simulink model "UFR_Monitoring_System"  (R2023a)
settings: Solver=VariableStepAuto  StartTime=0.0  StopTime=3600*4  RelTol=1e-3
undefined symbols (not defined in the file): out
settings Model: PacingRate=0.100000  Creator=alibacon  LastModifiedBy=ppatel
settings DataIOCC: SaveOutput=off  SaveTime=off
settings DebuggingCC: SubsystemReferenceDiagnosticForUnitTest=warning

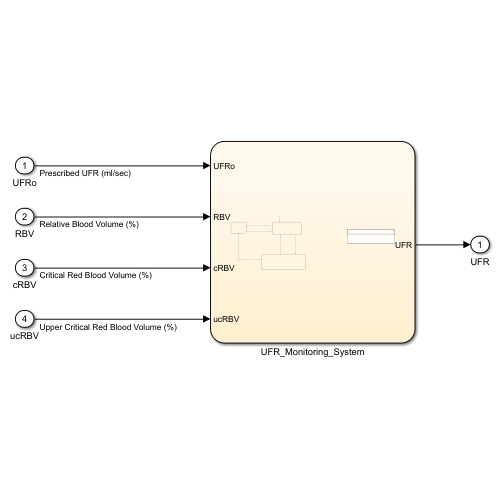
[thumbnail: Simulink's stored preview of the top-level diagram]
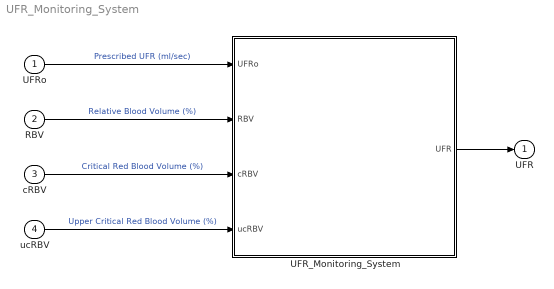
== system UFR_Monitoring_System ==
  UFRo : Inport  OutDataTypeStr=double  PortDimensions=1
  RBV : Inport  Port=2  OutDataTypeStr=double  PortDimensions=1  SampleTime=0
  cRBV : Inport  Port=3  OutDataTypeStr=double  PortDimensions=1  SampleTime=[0,1]
  ucRBV : Inport  Port=4  OutDataTypeStr=double  PortDimensions=1  SampleTime=[0,1]
  UFR_Monitoring_System : Stateflow chart  TreatAsAtomicUnit=on
  UFR : Outport  OutDataTypeStr=double  PortDimensions=1  SampleTime=[0,1]
  wires:
  UFRo/1 -> UFR_Monitoring_System/1(UFRo)  "Prescribed UFR (ml/sec)"
  RBV/1 -> UFR_Monitoring_System/2(RBV)  "Relative Blood Volume (%)"
  cRBV/1 -> UFR_Monitoring_System/3(cRBV)  "Critical Red Blood Volume (%)"
  ucRBV/1 -> UFR_Monitoring_System/4(ucRBV)  "Upper Critical Red Blood Volume (%)"
  UFR_Monitoring_System/1(UFR) -> UFR/1

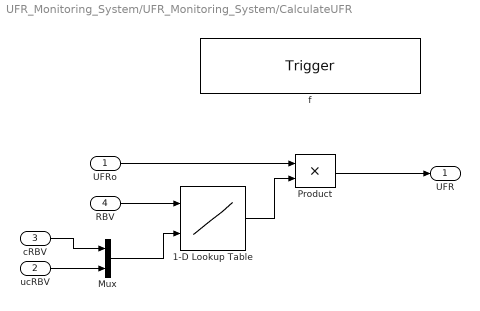
== system UFR_Monitoring_System/UFR_Monitoring_System/CalculateUFR ==
  UFRo : Inport  OutDataTypeStr=double  PortDimensions=1
  ucRBV : Inport  Port=2  OutDataTypeStr=double  PortDimensions=1
  cRBV : Inport  Port=3  OutDataTypeStr=double  PortDimensions=1
  RBV : Inport  Port=4  OutDataTypeStr=double  PortDimensions=1
  f : TriggerPort  TriggerType=function-call  VariantControl=(inherit)
      settings: CopyFcn=Stateflow.SLINSF.SimulinkMan.removeBlockPreDeleteFcn  PreDeleteFcn=Stateflow.SLINSF.SimulinkMan.unsafePredeleteFcn
  1-D Lookup Table : Lookup_n-D  NumberOfTableDimensions=1  BreakpointsForDimension1Source=Input port  BreakpointsForDimension1=[out.cRBV out.ucRBV]  Table=[0 1]  InternalRulePriority=Speed  RndMeth=Simplest
      settings: InputPortMap=u0,p5
  Mux : Mux  Inputs=2
  Product : Product
  UFR : Outport
  wires:
  RBV/1 -> 1-D Lookup Table/1
  cRBV/1 -> Mux/1
  UFRo/1 -> Product/1
  Mux/1 -> 1-D Lookup Table/2
  ucRBV/1 -> Mux/2
  1-D Lookup Table/1 -> Product/2
  Product/1 -> UFR/1

== stateflow chart UFR_Monitoring_System/UFR_Monitoring_System ==
  state Stop
    UFR=0;
  state NoCalc
    UFR=UFRo;
  state UFR = CalculateUFR(UFRo,ucRBV,cRBV,RBV) [function]
  state ReCalc
    UFR = CalculateUFR(UFRo,ucRBV,cRBV,RBV);
  (default) -> NoCalc
  NoCalc -> Stop [order 2] : [RBV <= cRBV]
  Stop -> NoCalc : [RBV > cRBV]
  (junction 68) -> Stop
  ReCalc -> NoCalc [order 1] : [RBV >=ucRBV]
  NoCalc -> ReCalc [order 1] : [(RBV > cRBV) && (RBV < ucRBV)]
  ReCalc -> (junction 68) [order 2] : [RBV <= cRBV]
  data: UFRo function_input double size=1; ucRBV function_input double size=1; cRBV function_input double size=1; RBV function_input double size=1; UFR function_output; UFRo input; RBV input; cRBV input; UFR output; ucRBV input
